simulink model "Energy_sim"  (R2025a)
settings: Solver=FixedStepAuto  StartTime=0.0  StopTime=1370  FixedStep=1  RelTol=1e-3
settings Model: Creator=user  LastModifiedBy=user
settings DataIOCC: SaveFinalState=on  SaveFormat=StructureWithTime  LoggingIntervals=[-inf,inf]
settings DebuggingCC: InheritedTsInSrcMsg=none

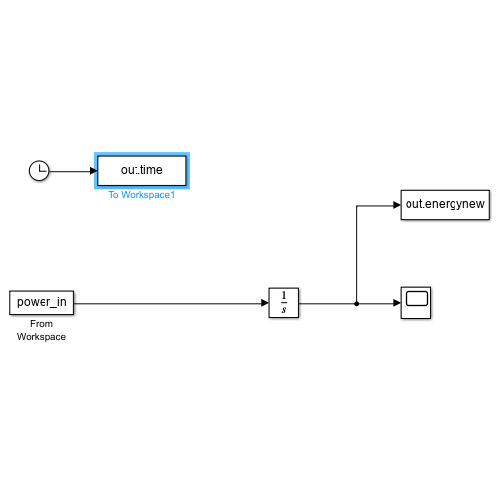
[thumbnail: Simulink's stored preview of the top-level diagram]
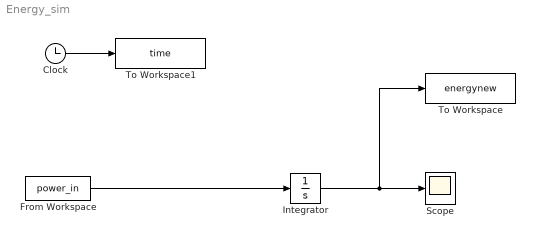
== system Energy_sim ==
  Clock : Clock
  From Workspace : FromWorkspace  VariableName=power_in  SampleTime=1  OutputAfterFinalValue=Holding final value
  Integrator : Integrator
  Scope : Scope
      settings: ActiveDisplayYMinimum=-8.63807524642E+6  ActiveDisplayYMaximum=7.774267721778E+7
  To Workspace : ToWorkspace  VariableName=energynew  SampleTime=-1
      settings: Save2DSignal=2-D array (concatenate along first dimension)
  To Workspace1 : ToWorkspace  VariableName=time  SampleTime=-1
      settings: Save2DSignal=2-D array (concatenate along first dimension)
  wires:
  Integrator/1 -> To Workspace/1, Scope/1
  From Workspace/1 -> Integrator/1
  Clock/1 -> To Workspace1/1
